simulink model "Test2_feedback_linearization_control"  (R2022b)
settings: Solver=VariableStepAuto  StartTime=0.0  StopTime=20.0  RelTol=1e-3
values from neighbouring files (symbols this model uses):
  g = 9.8    [config.m]
  Jx = 2*Mc*R^2/5 + 2*m*l^2    (= 0.0448)    [config.m]
  Jy = 2*Mc*R^2/5 + 2*m*l^2    (= 0.0448)    [config.m]
  Jz = 2*Mc*R^2/5 + 4*m*l^2    (= 0.0808)    [config.m]
  K_phi = 80    [config.m]
  K_psi = 80    [config.m]
  K_theta = 80    [config.m]
  K_z = 80    [config.m]
  Kd_pitch = 15    [config.m]
  Kd_roll = 15    [config.m]
  Kd_yaw = 15    [config.m]
  Kd_z = 15    [config.m]
  Ki_pitch = 1    [config.m]
  Ki_roll = 1    [config.m]
  Ki_yaw = 1    [config.m]
  Ki_z = 10    [config.m]
  Kp_pitch = 80    [config.m]
  Kp_roll = 80    [config.m]
  Kp_yaw = 80    [config.m]
  Kp_z = 80    [config.m]
  l = 0.3    [config.m]
  lumda_phi = 1    [config.m]
  lumda_psi = 1    [config.m]
  lumda_theta = 1    [config.m]
  lumda_z = 1    [config.m]
  M = Mc + 4*m    (= 3)    [config.m]
libraries: simulink x2
settings Model: Creator=cxk  LastModifiedBy=cxk

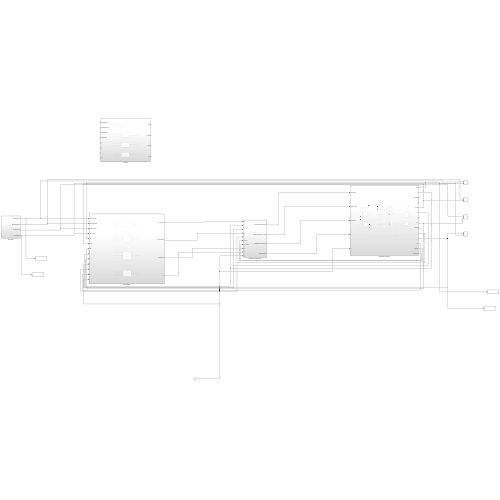
[thumbnail: Simulink's stored preview of the top-level diagram]
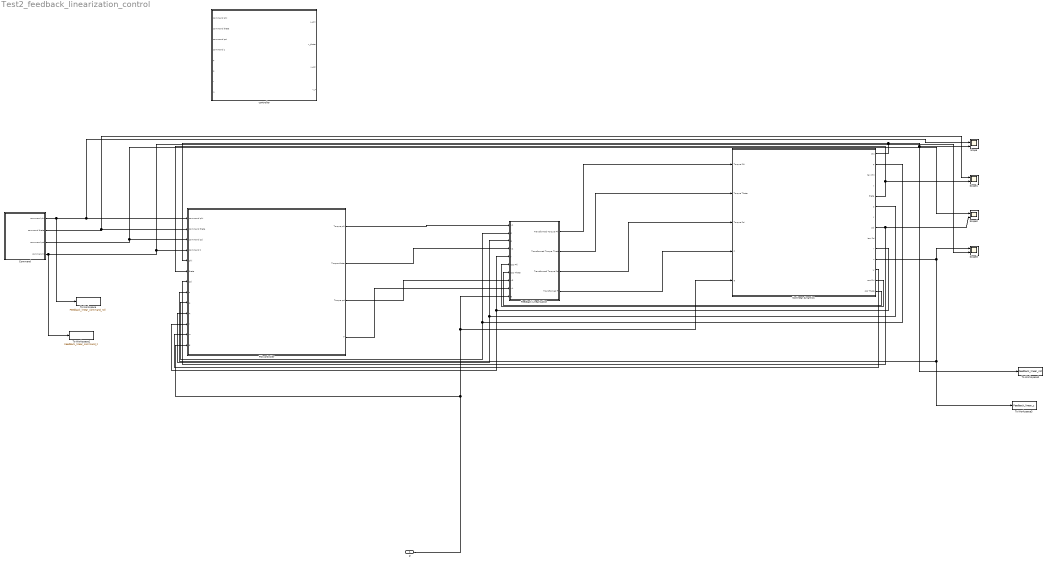
== system Test2_feedback_linearization_control ==
  g : Inport
  Command : Subsystem
  Feedback Linearization : Subsystem
  Nonlinear dynamics : Subsystem
  PID controller : Subsystem
  Scope{,1..3} (4 alike) : Scope  NumInputPorts=2
  To Workspace : ToWorkspace  VariableName=Feedback_linear_command_roll  SaveFormat=Timeseries  SampleTime=-1
  To Workspace1 : ToWorkspace  VariableName=Feedback_linear_command_z  SaveFormat=Timeseries  SampleTime=-1
  To Workspace2 : ToWorkspace  VariableName=Feedback_linear_roll  SaveFormat=Timeseries  SampleTime=-1
  To Workspace3 : ToWorkspace  VariableName=Feedback_linear_z  SaveFormat=Timeseries  SampleTime=-1
  controller : Subsystem
  wires:
  Nonlinear dynamics/2(p) -> PID controller/9(p), Feedback Linearization/2(p)
  Nonlinear dynamics/6(q) -> PID controller/10(q), Feedback Linearization/3(q)
  Nonlinear dynamics/10(r) -> PID controller/11(r), Feedback Linearization/5(r)
  Nonlinear dynamics/13(cos Phi) -> Feedback Linearization/6(cos Phi)
  Nonlinear dynamics/14(cos Theta) -> Feedback Linearization/7(cos Theta)
  Feedback Linearization/1(Transformed Torque Phi) -> Nonlinear dynamics/1(Torque Phi)
  Feedback Linearization/2(Transformed Torque Theta) -> Nonlinear dynamics/2(Torque Theta)
  Feedback Linearization/3(Transformed Torque Psi) -> Nonlinear dynamics/3(Torque Psi)
  Feedback Linearization/4(Transformed F) -> Nonlinear dynamics/4(F)
  g/1 -> PID controller/13(g), Nonlinear dynamics/5(g), Feedback Linearization/10(g)
  Nonlinear dynamics/5(theta) -> PID controller/6(theta), Scope1/2
  Nonlinear dynamics/8(psi) -> Scope2/2, PID controller/7(psi)
  Command/1(command phi) -> To Workspace/1, Scope/1, PID controller/1(command phi)
  Command/2(command theta) -> Scope1/1, PID controller/2(command theta)
  Command/3(command psi) -> Scope2/1, PID controller/3("command psi ")
  Command/4(command z) -> To Workspace1/1, Scope3/2, PID controller/4(command z)
  Nonlinear dynamics/12(w) -> PID controller/12(w)
  PID controller/1(Torque phi) -> Feedback Linearization/1(v1)
  PID controller/2(Torque theta) -> Feedback Linearization/4(v2)
  PID controller/3(Torque psi) -> Feedback Linearization/8(v3)
  PID controller/4(F) -> Feedback Linearization/9(v4)
  Nonlinear dynamics/11(z) -> To Workspace3/1, PID controller/8(z), Scope3/1
  Nonlinear dynamics/1(Phi) -> Scope/2, To Workspace2/1, PID controller/5(phi)

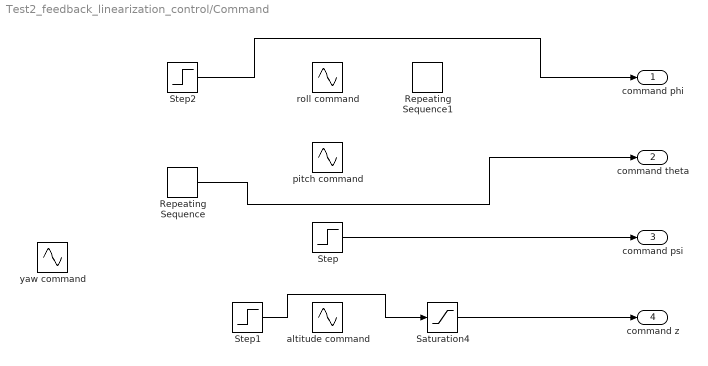
== system Test2_feedback_linearization_control/Command ==
  Repeating Sequence : simulink/Sources/Repeating Sequence  rep_seq_t="[0 1 1.01  3 3.01 4 4.01 6]"  rep_seq_y=[0 0 1 1 -1 -1 0 0 ]
  Repeating Sequence1 : simulink/Sources/Repeating Sequence  rep_seq_t="[0 2 2.01  4 4.01 5 5.01 6]"  rep_seq_y=[0 0 1 1 -1 -1 0 0 ]
  Saturation4 : Saturate  UpperLimit=5  LowerLimit=-5
  Step : Step  After=0  SampleTime=0
  Step1 : Step  After=-3  SampleTime=0
  Step2 : Step  After=0.68  SampleTime=0
  altitude command : Sin  Amplitude=10  Frequency=0.5  SampleTime=0
  pitch command : Sin  Amplitude=0.68  Frequency=0.5  SampleTime=0
  roll command : Sin  Amplitude=0.68  Frequency=0.5  SampleTime=0
  yaw command : Sin  Amplitude=pi  Frequency=0.5  SampleTime=0
  command phi : Outport
  command theta : Outport  Port=2
  command psi : Outport  Port=3
  command z : Outport  Port=4
  wires:
  Saturation4/1 -> command z/1
  Step/1 -> command psi/1
  Repeating Sequence/1 -> command theta/1
  Step1/1 -> Saturation4/1
  Step2/1 -> command phi/1

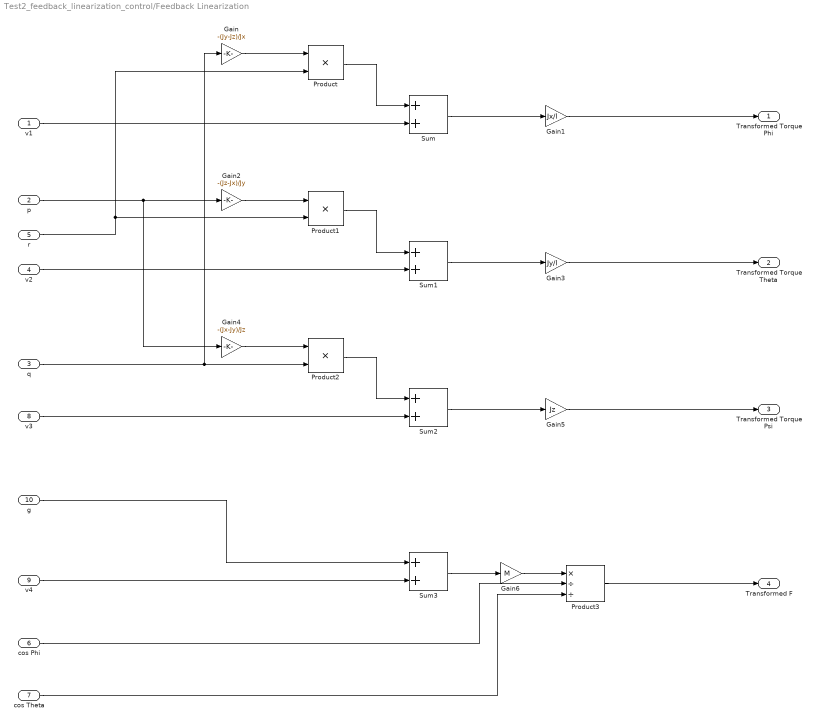
== system Test2_feedback_linearization_control/Feedback Linearization ==
  v1 : Inport
  p : Inport  Port=2
  q : Inport  Port=3
  v2 : Inport  Port=4
  r : Inport  Port=5
  cos Phi : Inport  Port=6
  cos Theta : Inport  Port=7
  v3 : Inport  Port=8
  v4 : Inport  Port=9
  g : Inport  Port=10
  Gain : Gain  Gain=-(Jy-Jz)/Jx
  Gain1 : Gain  Gain=Jx/l
  Gain2 : Gain  Gain=-(Jz-Jx)/Jy
  Gain3 : Gain  Gain=Jy/l
  Gain4 : Gain  Gain=-(Jx-Jy)/Jz
  Gain5 : Gain  Gain=Jz
  Gain6 : Gain  Gain=M
  Product : Product
  Product1 : Product
  Product2 : Product
  Product3 : Product  Inputs=*//
  Sum{,1..3} (4 alike) : Sum
  Transformed Torque Phi : Outport
  Transformed Torque Theta : Outport  Port=2
  Transformed Torque Psi : Outport  Port=3
  Transformed F : Outport  Port=4
  wires:
  Sum/1 -> Gain1/1
  Product1/1 -> Sum1/1
  Sum1/1 -> Gain3/1
  r/1 -> Product/2, Product1/2
  v2/1 -> Sum1/2
  g/1 -> Sum3/1
  Gain2/1 -> Product1/1
  Sum2/1 -> Gain5/1
  p/1 -> Gain4/1, Gain2/1
  cos Phi/1 -> Product3/2
  Product/1 -> Sum/1
  Sum3/1 -> Gain6/1
  v3/1 -> Sum2/2
  Gain/1 -> Product/1
  q/1 -> Gain/1, Product2/2
  v1/1 -> Sum/2
  cos Theta/1 -> Product3/3
  Gain6/1 -> Product3/1
  Gain3/1 -> Transformed Torque Theta/1
  Gain4/1 -> Product2/1
  Product2/1 -> Sum2/1
  v4/1 -> Sum3/2
  Product3/1 -> Transformed F/1
  Gain1/1 -> Transformed Torque Phi/1
  Gain5/1 -> Transformed Torque Psi/1

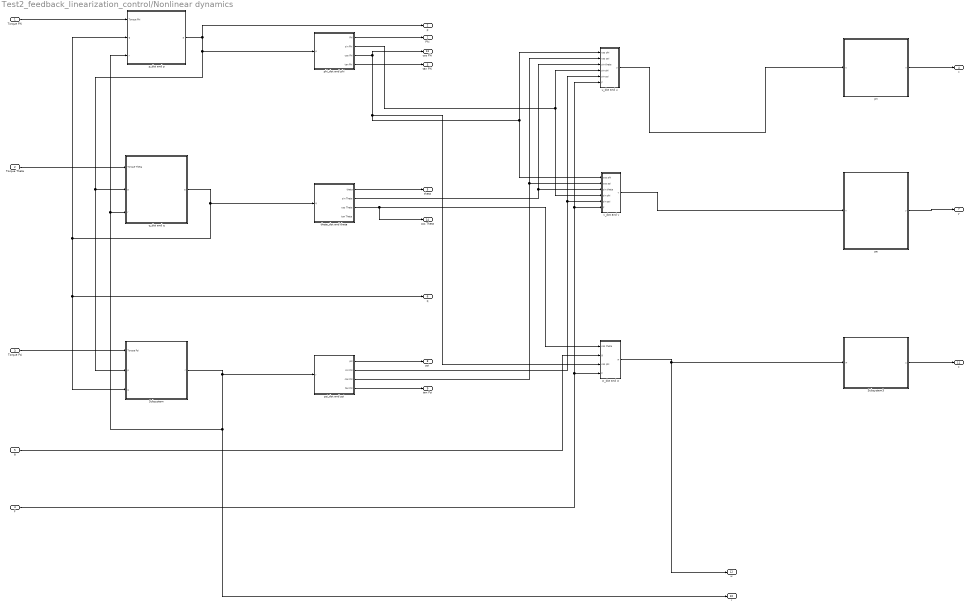
== system Test2_feedback_linearization_control/Nonlinear dynamics ==
  Torque Phi : Inport
  Torque Theta : Inport  Port=2
  Torque Psi : Inport  Port=3
  F : Inport  Port=4
  g : Inport  Port=5
  Subsystem : Subsystem
  Subsystem3 : Subsystem
  p_dot and p : Subsystem
  pe : Subsystem
  phi_dot and phi : Subsystem
  pn : Subsystem
  psi_dot and psi : Subsystem
  q_dot and q : Subsystem
  theta_dot and theta : Subsystem
  u_dot and u : Subsystem
  v_dot and v : Subsystem
  w_dot and w : Subsystem
  Phi : Outport
  p : Outport  Port=2
  tan Phi : Outport  Port=3
  x : Outport  Port=4
  theta : Outport  Port=5
  q : Outport  Port=6
  y : Outport  Port=7
  psi : Outport  Port=8
  tan Psi : Outport  Port=9
  r : Outport  Port=10
  z : Outport  Port=11
  w : Outport  Port=12
  cos Phi : Outport  Port=13
  cos Theta : Outport  Port=14
  wires:
  psi_dot and psi/3(cos Psi) -> u_dot and u/2(cos psi), v_dot and v/2(cos psi)
  phi_dot and phi/3(cos Phi) -> cos Phi/1, v_dot and v/1(cos phi), u_dot and u/1(cos phi), w_dot and w/3(cos phi)
  theta_dot and theta/3(cos Theta) -> cos Theta/1, w_dot and w/1(cos theta)
  u_dot and u/1(u) -> pn/1(u)
  w_dot and w/1(w) -> w/1, Subsystem3/1(w)
  g/1 -> w_dot and w/2(g)
  theta_dot and theta/2(sin Theta) -> v_dot and v/3(sin theta), u_dot and u/3(sin theta)
  q_dot and q/1(q) -> q/1, Subsystem/3(q), p_dot and p/2(q), theta_dot and theta/1(q)
  phi_dot and phi/2(sin Phi) -> v_dot and v/4(sin phi), u_dot and u/4(sin phi)
  v_dot and v/1(v) -> pe/1(v)
  Torque Theta/1 -> q_dot and q/1(Torque Theta)
  psi_dot and psi/2(sin Psi) -> v_dot and v/5(sin psi), u_dot and u/5(sin psi)
  p_dot and p/1(p) -> q_dot and q/2(p), Subsystem/2(p), phi_dot and phi/1(p), p/1
  pn/1(x) -> x/1
  theta_dot and theta/1(theta) -> theta/1
  Subsystem/1(r) -> psi_dot and psi/1(r), p_dot and p/3(r), q_dot and q/3(r), r/1
  psi_dot and psi/1(psi) -> psi/1
  Torque Phi/1 -> p_dot and p/1(Torque Phi)
  Torque Psi/1 -> Subsystem/1(Torque Psi)
  phi_dot and phi/1(Phi) -> Phi/1
  psi_dot and psi/4(tan Psi) -> tan Psi/1
  phi_dot and phi/4(tan Phi) -> tan Phi/1
  pe/1(y) -> y/1
  Subsystem3/1(z) -> z/1
  F/1 -> w_dot and w/4(F), v_dot and v/6(F), u_dot and u/6(F)

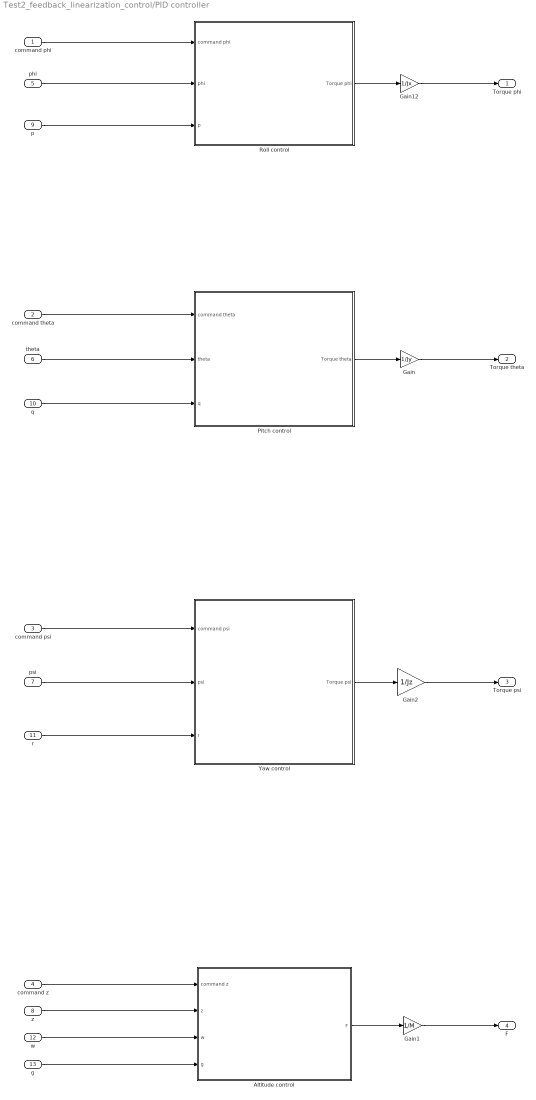
== system Test2_feedback_linearization_control/PID controller ==
  command phi : Inport
  command theta : Inport  Port=2
  "command psi " : Inport  Port=3
  command z : Inport  Port=4
  phi : Inport  Port=5
  theta : Inport  Port=6
  psi : Inport  Port=7
  z : Inport  Port=8
  p : Inport  Port=9
  q : Inport  Port=10
  r : Inport  Port=11
  w : Inport  Port=12
  g : Inport  Port=13
  Altitude control : Subsystem
  Gain : Gain  Gain=1/Jy
  Gain1 : Gain  Gain=1/M
  Gain12 : Gain  Gain=1/Jx
  Gain2 : Gain  Gain=1/Jz
  Pitch control : Subsystem
  Roll control : Subsystem
  Yaw control : Subsystem
  Torque phi : Outport
  Torque theta : Outport  Port=2
  Torque psi : Outport  Port=3
  F : Outport  Port=4
  wires:
  phi/1 -> Roll control/2(phi)
  command phi/1 -> Roll control/1(command phi)
  theta/1 -> Pitch control/2(theta)
  command theta/1 -> Pitch control/1(command theta)
  command z/1 -> Altitude control/1(command z)
  Yaw control/1(Torque psi) -> Gain2/1
  z/1 -> Altitude control/2(z)
  "command psi "/1 -> Yaw control/1("command psi ")
  w/1 -> Altitude control/3(w)
  q/1 -> Pitch control/3(q)
  Altitude control/1(F) -> Gain1/1
  Pitch control/1(Torque theta) -> Gain/1
  psi/1 -> Yaw control/2(psi)
  Roll control/1(Torque phi) -> Gain12/1
  r/1 -> Yaw control/3(r)
  p/1 -> Roll control/3(p)
  g/1 -> Altitude control/4(g)
  Gain2/1 -> Torque psi/1
  Gain/1 -> Torque theta/1
  Gain12/1 -> Torque phi/1
  Gain1/1 -> F/1

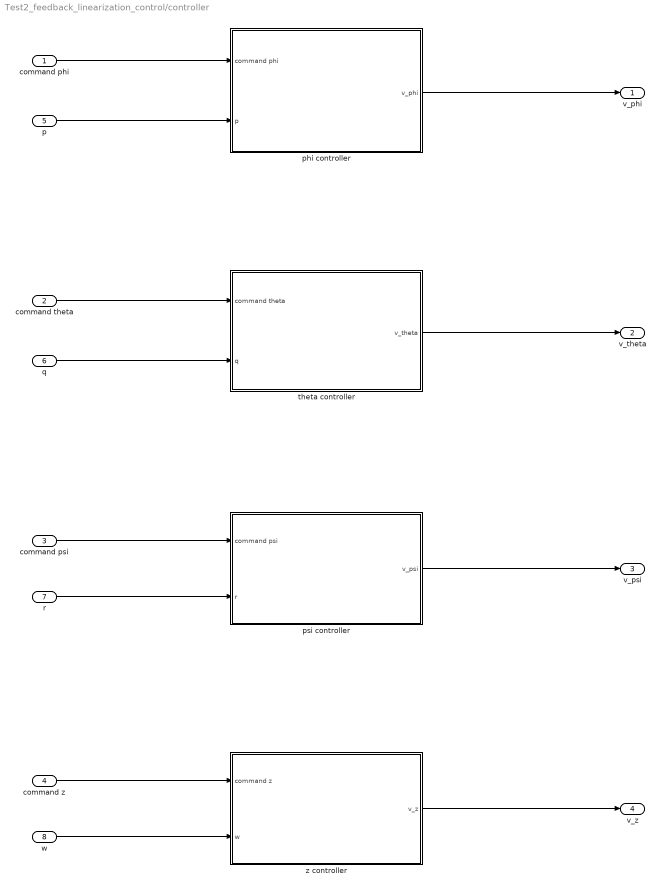
== system Test2_feedback_linearization_control/controller ==
  command phi : Inport
  command theta : Inport  Port=2
  command psi : Inport  Port=3
  command z : Inport  Port=4
  p : Inport  Port=5
  q : Inport  Port=6
  r : Inport  Port=7
  w : Inport  Port=8
  phi controller : Subsystem
  psi controller : Subsystem
  theta controller : Subsystem
  z controller : Subsystem
  v_phi : Outport
  v_theta : Outport  Port=2
  v_psi : Outport  Port=3
  v_z : Outport  Port=4
  wires:
  command phi/1 -> phi controller/1(command phi)
  phi controller/1(v_phi) -> v_phi/1
  command theta/1 -> theta controller/1(command theta)
  theta controller/1(v_theta) -> v_theta/1
  command psi/1 -> psi controller/1(command psi)
  psi controller/1(v_psi) -> v_psi/1
  command z/1 -> z controller/1(command z)
  z controller/1(v_z) -> v_z/1
  p/1 -> phi controller/2(p)
  q/1 -> theta controller/2(q)
  r/1 -> psi controller/2(r)
  w/1 -> z controller/2(w)

== system Test2_feedback_linearization_control/Nonlinear dynamics/Subsystem ==
  note: $\dot r$
  note: ${(J_x-J_y) \over J_z}pq$
  note: r_dot and r
  note: $r$
  Torque Psi : Inport
  p : Inport  Port=2
  q : Inport  Port=3
  Gain2 : Gain  Gain=1/Jz
  Gain20 : Gain  Gain=(Jx-Jy)/Jz
  Integrator4 : Integrator
  Product2 : Product
  Sum11 : Sum
  r : Outport
  wires:
  Gain20/1 -> Product2/1
  Torque Psi/1 -> Gain2/1
  p/1 -> Gain20/1
  Sum11/1 -> Integrator4/1
  Product2/1 -> Sum11/2
  q/1 -> Product2/2
  Integrator4/1 -> r/1
  Gain2/1 -> Sum11/1

== system Test2_feedback_linearization_control/Nonlinear dynamics/Subsystem3 ==
  note: $h$
  note: $\dot h$
  w : Inport
  Integrator : Integrator
  z : Outport
  wires:
  w/1 -> Integrator/1
  Integrator/1 -> z/1

== system Test2_feedback_linearization_control/Nonlinear dynamics/p_dot and p ==
  note: p_dot and p
  note: ${(J_y-J_z) \over J_x}qr$
  note: $\dot p$
  note: $p$
  Torque Phi : Inport
  q : Inport  Port=2
  r : Inport  Port=3
  Gain12 : Gain  Gain=1/Jx
  Gain17 : Gain  Gain=(Jy-Jz)/Jx
  Integrator2 : Integrator
  Product : Product
  Sum9 : Sum
  p : Outport
  wires:
  Sum9/1 -> Integrator2/1
  Product/1 -> Sum9/2
  r/1 -> Product/2
  Integrator2/1 -> p/1
  Gain17/1 -> Product/1
  Gain12/1 -> Sum9/1
  Torque Phi/1 -> Gain12/1
  q/1 -> Gain17/1

== system Test2_feedback_linearization_control/Nonlinear dynamics/pe ==
  note: $\dot p_e$
  note: $p_e$
  v : Inport
  Integrator : Integrator
  y : Outport
  wires:
  v/1 -> Integrator/1
  Integrator/1 -> y/1

== system Test2_feedback_linearization_control/Nonlinear dynamics/phi_dot and phi ==
  note: $\phi$
  note: $\dot \phi$
  p : Inport
  Integrator1 : Integrator
  Subsystem1 : Subsystem
  Phi : Outport
  sin Phi : Outport  Port=2
  cos Phi : Outport  Port=3
  tan Phi : Outport  Port=4
  wires:
  Subsystem1/2(cos Phi) -> cos Phi/1
  Subsystem1/1(sin Phi) -> sin Phi/1
  Integrator1/1 -> Phi/1, Subsystem1/1(phi)
  p/1 -> Integrator1/1
  Subsystem1/3(tan Phi) -> tan Phi/1

== system Test2_feedback_linearization_control/Nonlinear dynamics/pn ==
  note: $\dot p_n$
  note: $p_n$
  u : Inport
  Integrator : Integrator
  x : Outport
  wires:
  u/1 -> Integrator/1
  Integrator/1 -> x/1

== system Test2_feedback_linearization_control/Nonlinear dynamics/psi_dot and psi ==
  note: $\Psi$
  note: $\dot \Psi$
  r : Inport
  Integrator4 : Integrator
  Subsystem2 : Subsystem
  psi : Outport
  sin Psi : Outport  Port=2
  cos Psi : Outport  Port=3
  tan Psi : Outport  Port=4
  wires:
  Subsystem2/2(cos Psi) -> cos Psi/1
  r/1 -> Integrator4/1
  Integrator4/1 -> psi/1, Subsystem2/1(psi)
  Subsystem2/1(sin Psi) -> sin Psi/1
  Subsystem2/3(tan Psi) -> tan Psi/1

== system Test2_feedback_linearization_control/Nonlinear dynamics/q_dot and q ==
  note: $\dot q$
  note: ${(J_z-J_x) \over J_y}pr$
  note: q_dot and q
  note: $q$
  Torque Theta : Inport
  p : Inport  Port=2
  r : Inport  Port=3
  Gain16 : Gain  Gain=1/Jy
  Gain19 : Gain  Gain=(Jz-Jx)/Jy
  Integrator1 : Integrator
  Product1 : Product
  Sum10 : Sum
  q : Outport
  wires:
  Gain16/1 -> Sum10/1
  Integrator1/1 -> q/1
  Sum10/1 -> Integrator1/1
  r/1 -> Product1/2
  Gain19/1 -> Product1/1
  Product1/1 -> Sum10/2
  Torque Theta/1 -> Gain16/1
  p/1 -> Gain19/1

== system Test2_feedback_linearization_control/Nonlinear dynamics/theta_dot and theta ==
  note: $\theta$
  note: $\dot \theta$
  q : Inport
  Integrator2 : Integrator
  Subsystem2 : Subsystem
  theta : Outport
  sin Theta : Outport  Port=2
  cos Theta : Outport  Port=3
  tan Theta : Outport  Port=4
  wires:
  Subsystem2/1(sin Theta) -> sin Theta/1
  q/1 -> Integrator2/1
  Integrator2/1 -> theta/1, Subsystem2/1(theta)
  Subsystem2/3(tan Theta) -> tan Theta/1
  Subsystem2/2(cos Theta) -> cos Theta/1

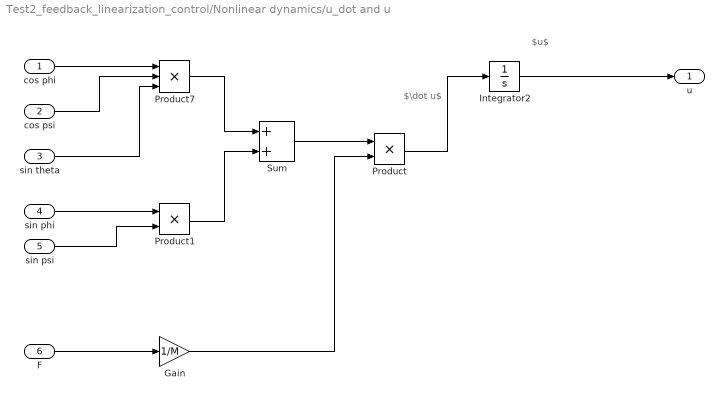
== system Test2_feedback_linearization_control/Nonlinear dynamics/u_dot and u ==
  note: $\dot u$
  note: $u$
  cos phi : Inport
  cos psi : Inport  Port=2
  sin theta : Inport  Port=3
  sin phi : Inport  Port=4
  sin psi : Inport  Port=5
  F : Inport  Port=6
  Gain : Gain  Gain=1/M
  Integrator2 : Integrator
  Product : Product
  Product1 : Product
  Product7 : Product  Inputs=3
  Sum : Sum
  u : Outport
  wires:
  Sum/1 -> Product/1
  Product/1 -> Integrator2/1
  Gain/1 -> Product/2
  Product7/1 -> Sum/1
  sin theta/1 -> Product7/3
  cos phi/1 -> Product7/1
  Product1/1 -> Sum/2
  F/1 -> Gain/1
  sin phi/1 -> Product1/1
  cos psi/1 -> Product7/2
  sin psi/1 -> Product1/2
  Integrator2/1 -> u/1

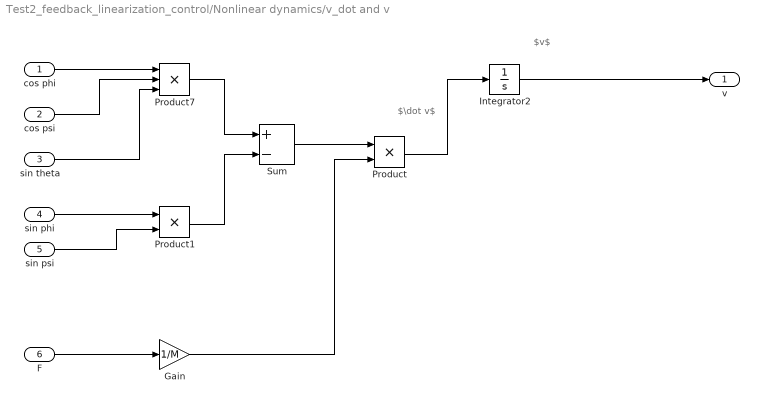
== system Test2_feedback_linearization_control/Nonlinear dynamics/v_dot and v ==
  note: $\dot v$
  note: $v$
  cos phi : Inport
  cos psi : Inport  Port=2
  sin theta : Inport  Port=3
  sin phi : Inport  Port=4
  sin psi : Inport  Port=5
  F : Inport  Port=6
  Gain : Gain  Gain=1/M
  Integrator2 : Integrator
  Product : Product
  Product1 : Product
  Product7 : Product  Inputs=3
  Sum : Sum  Inputs=+-
  v : Outport
  wires:
  cos phi/1 -> Product7/1
  Integrator2/1 -> v/1
  cos psi/1 -> Product7/2
  sin theta/1 -> Product7/3
  Sum/1 -> Product/1
  sin phi/1 -> Product1/1
  sin psi/1 -> Product1/2
  F/1 -> Gain/1
  Gain/1 -> Product/2
  Product7/1 -> Sum/1
  Product1/1 -> Sum/2
  Product/1 -> Integrator2/1

== system Test2_feedback_linearization_control/Nonlinear dynamics/w_dot and w ==
  note: $\dot w$
  note: $w$
  cos theta : Inport
  g : Inport  Port=2
  cos phi : Inport  Port=3
  F : Inport  Port=4
  Gain : Gain  Gain=1/M
  Integrator4 : Integrator
  Product8 : Product  Inputs=3
  Sum11 : Sum  Inputs=-+
  w : Outport
  wires:
  cos phi/1 -> Product8/3
  Product8/1 -> Sum11/2
  Sum11/1 -> Integrator4/1
  Integrator4/1 -> w/1
  g/1 -> Sum11/1
  cos theta/1 -> Product8/1
  F/1 -> Gain/1
  Gain/1 -> Product8/2

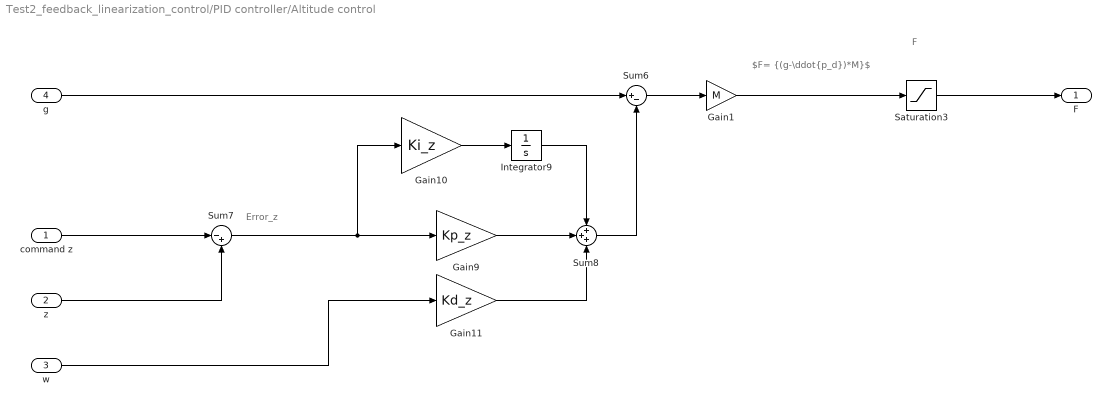
== system Test2_feedback_linearization_control/PID controller/Altitude control ==
  note: $F= {(g-\ddot{p_d})*M}$
  note: Error_z
  note: F
  command z : Inport
  z : Inport  Port=2
  w : Inport  Port=3
  g : Inport  Port=4
  Gain1 : Gain  Gain=M
  Gain10 : Gain  Gain=Ki_z
  Gain11 : Gain  Gain=Kd_z
  Gain9 : Gain  Gain=Kp_z
  Integrator9 : Integrator
  Saturation3 : Saturate  UpperLimit=g*M*10  LowerLimit=-2.97*M*10
  Sum6 : Sum  Inputs=|+-
  Sum7 : Sum  Inputs=|-+
  Sum8 : Sum  Inputs=+++
  F : Outport
  wires:
  Sum6/1 -> Gain1/1
  Sum7/1 -> Gain10/1, Gain9/1
  Gain9/1 -> Sum8/2
  Integrator9/1 -> Sum8/1
  g/1 -> Sum6/1
  Gain10/1 -> Integrator9/1
  Sum8/1 -> Sum6/2
  Gain1/1 -> Saturation3/1
  command z/1 -> Sum7/1
  Gain11/1 -> Sum8/3
  Saturation3/1 -> F/1
  z/1 -> Sum7/2
  w/1 -> Gain11/1

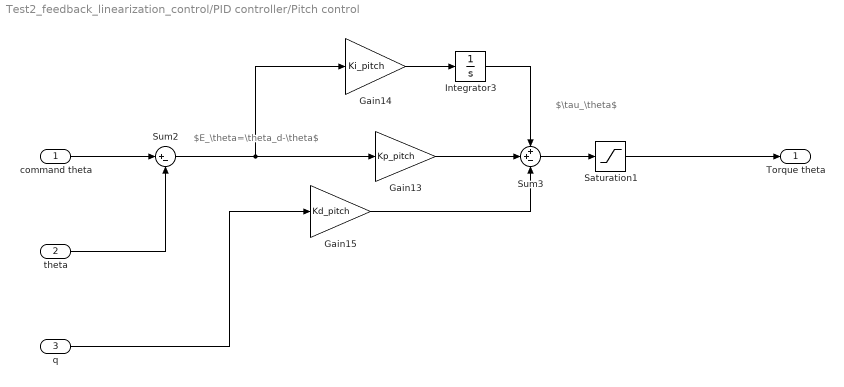
== system Test2_feedback_linearization_control/PID controller/Pitch control ==
  note: $E_\theta=\theta_d-\theta$
  note: $\tau_\theta$
  command theta : Inport
  theta : Inport  Port=2
  q : Inport  Port=3
  Gain13 : Gain  Gain=Kp_pitch
  Gain14 : Gain  Gain=Ki_pitch
  Gain15 : Gain  Gain=Kd_pitch
  Integrator3 : Integrator
  Saturation1 : Saturate  UpperLimit=100  LowerLimit=-100
  Sum2 : Sum  Inputs=|+-
  Sum3 : Sum  Inputs=++-
  Torque theta : Outport
  wires:
  command theta/1 -> Sum2/1
  Sum2/1 -> Gain14/1, Gain13/1
  Gain14/1 -> Integrator3/1
  Sum3/1 -> Saturation1/1
  Integrator3/1 -> Sum3/1
  Gain15/1 -> Sum3/3
  theta/1 -> Sum2/2
  Gain13/1 -> Sum3/2
  Saturation1/1 -> Torque theta/1
  q/1 -> Gain15/1

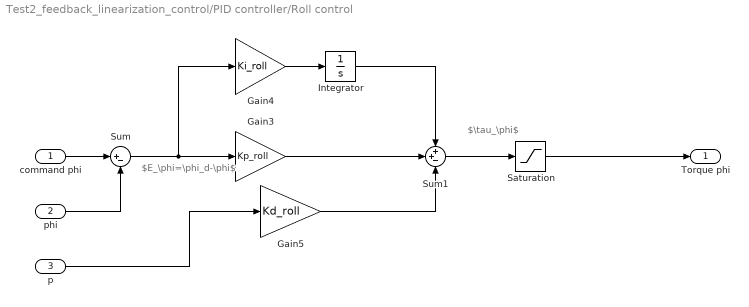
== system Test2_feedback_linearization_control/PID controller/Roll control ==
  note: $\tau_\phi$
  note: $E_\phi=\phi_d-\phi$
  command phi : Inport
  phi : Inport  Port=2
  p : Inport  Port=3
  Gain3 : Gain  Gain=Kp_roll
  Gain4 : Gain  Gain=Ki_roll
  Gain5 : Gain  Gain=Kd_roll
  Integrator : Integrator
  Saturation : Saturate  UpperLimit=100  LowerLimit=-100
  Sum : Sum  Inputs=|+-
  Sum1 : Sum  Inputs=++-
  Torque phi : Outport
  wires:
  Integrator/1 -> Sum1/1
  Sum/1 -> Gain4/1, Gain3/1
  Gain4/1 -> Integrator/1
  Gain5/1 -> Sum1/3
  Saturation/1 -> Torque phi/1
  Sum1/1 -> Saturation/1
  Gain3/1 -> Sum1/2
  command phi/1 -> Sum/1
  phi/1 -> Sum/2
  p/1 -> Gain5/1

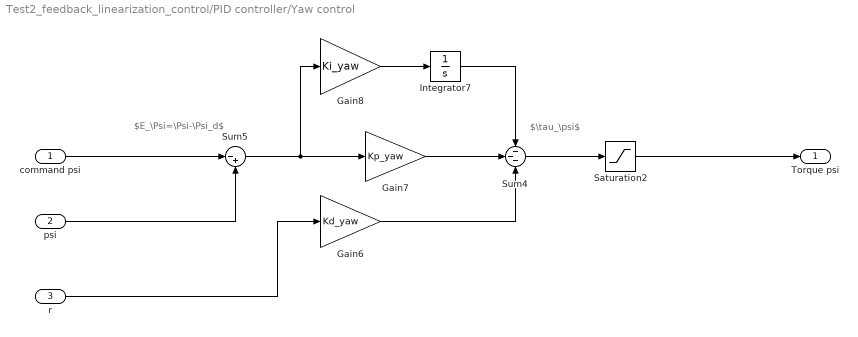
== system Test2_feedback_linearization_control/PID controller/Yaw control ==
  note: $E_\Psi=\Psi-\Psi_d$
  note: $\tau_\psi$
  "command psi " : Inport
  psi : Inport  Port=2
  r : Inport  Port=3
  Gain6 : Gain  Gain=Kd_yaw
  Gain7 : Gain  Gain=Kp_yaw
  Gain8 : Gain  Gain=Ki_yaw
  Integrator7 : Integrator
  Saturation2 : Saturate  UpperLimit=100  LowerLimit=-100
  Sum4 : Sum  Inputs=---
  Sum5 : Sum  Inputs=|-+
  Torque psi : Outport
  wires:
  Sum4/1 -> Saturation2/1
  Integrator7/1 -> Sum4/1
  Gain8/1 -> Integrator7/1
  psi/1 -> Sum5/2
  Sum5/1 -> Gain8/1, Gain7/1
  Gain7/1 -> Sum4/2
  Gain6/1 -> Sum4/3
  "command psi "/1 -> Sum5/1
  Saturation2/1 -> Torque psi/1
  r/1 -> Gain6/1

== system Test2_feedback_linearization_control/controller/phi controller ==
  note: $E_\phi=\dot \phi_d-\dot \phi$
  command phi : Inport
  p : Inport  Port=2
  Derivative : Derivative
  Derivative1 : Derivative
  Gain : Gain  Gain=-1/lumda_phi
  Gain1 : Gain  Gain=K_phi
  Integrator4 : Integrator
  Sum : Sum  Inputs=+-
  Sum1 : Sum  Inputs=+-+
  v_phi : Outport
  wires:
  Derivative1/1 -> Sum1/1
  Sum1/1 -> v_phi/1
  command phi/1 -> Derivative/1
  Derivative/1 -> Sum/1, Derivative1/1
  Sum/1 -> Gain1/1, Gain/1
  Gain1/1 -> Sum1/3
  p/1 -> Sum/2
  Integrator4/1 -> Sum1/2
  Gain/1 -> Integrator4/1

== system Test2_feedback_linearization_control/controller/psi controller ==
  note: $E_\psi=\dot \psi_d-\dot \psi$
  command psi : Inport
  r : Inport  Port=2
  Derivative4 : Derivative
  Derivative5 : Derivative
  Gain4 : Gain  Gain=-1/lumda_psi
  Gain5 : Gain  Gain=K_psi
  Integrator2 : Integrator
  Sum4 : Sum  Inputs=+-
  Sum5 : Sum  Inputs=+-+
  v_psi : Outport
  wires:
  Derivative4/1 -> Sum4/1, Derivative5/1
  Gain5/1 -> Sum5/3
  Sum4/1 -> Gain5/1, Gain4/1
  r/1 -> Sum4/2
  Integrator2/1 -> Sum5/2
  Sum5/1 -> v_psi/1
  Gain4/1 -> Integrator2/1
  command psi/1 -> Derivative4/1
  Derivative5/1 -> Sum5/1

== system Test2_feedback_linearization_control/controller/theta controller ==
  note: $E_\theta=\dot \theta_d-\dot \theta$
  command theta : Inport
  q : Inport  Port=2
  Derivative2 : Derivative
  Derivative3 : Derivative
  Gain2 : Gain  Gain=-1/lumda_theta
  Gain3 : Gain  Gain=K_theta
  Integrator6 : Integrator
  Sum2 : Sum  Inputs=+-
  Sum3 : Sum  Inputs=+-+
  v_theta : Outport
  wires:
  Derivative2/1 -> Sum2/1, Derivative3/1
  Sum3/1 -> v_theta/1
  Sum2/1 -> Gain3/1, Gain2/1
  q/1 -> Sum2/2
  Derivative3/1 -> Sum3/1
  Gain3/1 -> Sum3/3
  Gain2/1 -> Integrator6/1
  Integrator6/1 -> Sum3/2
  command theta/1 -> Derivative2/1

== system Test2_feedback_linearization_control/controller/z controller ==
  note: $E_z=\dot z_d-\dot z$
  command z : Inport
  w : Inport  Port=2
  Derivative6 : Derivative
  Derivative7 : Derivative
  Gain6 : Gain  Gain=-1/lumda_z
  Gain7 : Gain  Gain=K_z
  Integrator7 : Integrator
  Sum6 : Sum  Inputs=+-
  Sum7 : Sum  Inputs=+-+
  v_z : Outport
  wires:
  Sum6/1 -> Gain7/1, Gain6/1
  Integrator7/1 -> Sum7/2
  Gain6/1 -> Integrator7/1
  Gain7/1 -> Sum7/3
  Derivative7/1 -> Sum7/1
  Derivative6/1 -> Sum6/1, Derivative7/1
  w/1 -> Sum6/2
  Sum7/1 -> v_z/1
  command z/1 -> Derivative6/1

== system Test2_feedback_linearization_control/Nonlinear dynamics/phi_dot and phi/Subsystem1 ==
  phi : Inport
  Trigonometric Function : Trigonometry
  Trigonometric Function1 : Trigonometry  Operator=cos
  Trigonometric Function2 : Trigonometry  Operator=tan
  sin Phi : Outport
  cos Phi : Outport  Port=2
  tan Phi : Outport  Port=3
  wires:
  phi/1 -> Trigonometric Function2/1, Trigonometric Function1/1, Trigonometric Function/1
  Trigonometric Function2/1 -> tan Phi/1
  Trigonometric Function/1 -> sin Phi/1
  Trigonometric Function1/1 -> cos Phi/1

== system Test2_feedback_linearization_control/Nonlinear dynamics/psi_dot and psi/Subsystem2 ==
  psi : Inport
  Trigonometric Function : Trigonometry
  Trigonometric Function1 : Trigonometry  Operator=cos
  Trigonometric Function2 : Trigonometry  Operator=tan
  sin Psi : Outport
  cos Psi : Outport  Port=2
  tan Psi : Outport  Port=3
  wires:
  psi/1 -> Trigonometric Function2/1, Trigonometric Function1/1, Trigonometric Function/1
  Trigonometric Function2/1 -> tan Psi/1
  Trigonometric Function/1 -> sin Psi/1
  Trigonometric Function1/1 -> cos Psi/1

== system Test2_feedback_linearization_control/Nonlinear dynamics/theta_dot and theta/Subsystem2 ==
  theta : Inport
  Trigonometric Function : Trigonometry
  Trigonometric Function1 : Trigonometry  Operator=cos
  Trigonometric Function2 : Trigonometry  Operator=tan
  sin Theta : Outport
  cos Theta : Outport  Port=2
  tan Theta : Outport  Port=3
  wires:
  theta/1 -> Trigonometric Function2/1, Trigonometric Function1/1, Trigonometric Function/1
  Trigonometric Function2/1 -> tan Theta/1
  Trigonometric Function/1 -> sin Theta/1
  Trigonometric Function1/1 -> cos Theta/1
